simulink model "3Phase_Differential_Buck_Inverter"  (R2022b)
settings: Solver=VariableStepAuto  StartTime=0.0  StopTime=10.0  RelTol=1e-3
model workspace (MAT data in the model file):
  phi1 = 1.5991904307
  phi2 = 6.28
  phi3 = 3.23480337931
libraries: spsSeriesRLCBranchLib x9, spsGroundLib x7, spsMosfetLib x6, spsVoltageMeasurementLib x6, spsDCVoltageSourceLib x1, spsTriangleGeneratorLib x1, sps_lib x1
settings Model: Creator=nishi  LastModifiedBy=nishi

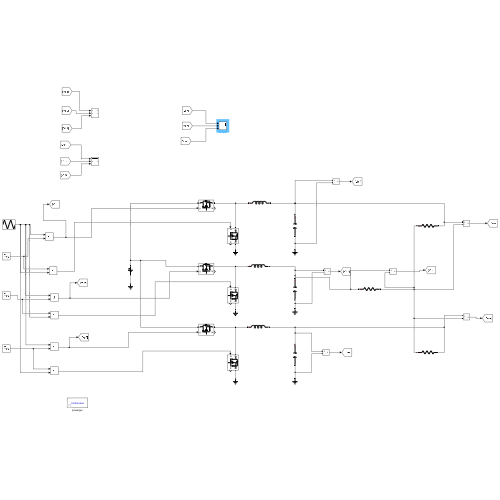
[thumbnail: Simulink's stored preview of the top-level diagram]
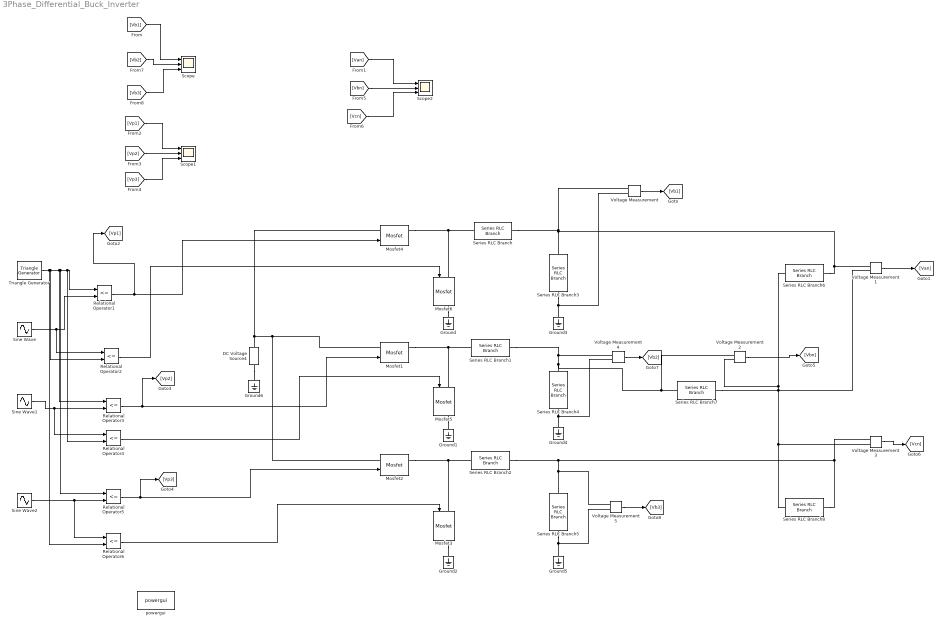
== system 3Phase_Differential_Buck_Inverter ==
  DC Voltage Source4 : spsDCVoltageSourceLib/DC Voltage Source  Amplitude=24  Measurements=None
  Ground{,1..6} (7 alike) : spsGroundLib/Ground  LConnTagsString=a
  Mosfet{1..6} (6 alike) : spsMosfetLib/Mosfet  Ron=1e-7  Lon=0  Rd=1e-10  Vfd=0  IC=0  Rs=inf  Cs=0  Measurements=on
  Relational Operator{1..6} (6 alike) : RelationalOperator  Operator=<=  OutDataTypeStr=boolean  RndMeth=Simplest  InputSameDT=off
  Scope : Scope  NumInputPorts=3
  Scope1 : Scope  NumInputPorts=3
  Scope2 : Scope  NumInputPorts=3
  Series RLC Branch : spsSeriesRLCBranchLib/Series RLC Branch  LConnTagsString=__new0  RConnTagsString=__new0  BranchType=L  Resistance=1  Inductance=3e-3  SetiL0=off  InitialCurrent=0  Capacitance=1e-6  Setx0=off  InitialVoltage=0  Measurements=None
  Series RLC Branch1 : spsSeriesRLCBranchLib/Series RLC Branch  LConnTagsString=__new0  RConnTagsString=__new0  BranchType=L  Resistance=1  Inductance=3e-3  SetiL0=off  InitialCurrent=0  Capacitance=1e-6  Setx0=off  InitialVoltage=0  Measurements=None
  Series RLC Branch2 : spsSeriesRLCBranchLib/Series RLC Branch  LConnTagsString=__new0  RConnTagsString=__new0  BranchType=L  Resistance=1  Inductance=3e-3  SetiL0=off  InitialCurrent=0  Capacitance=1e-6  Setx0=off  InitialVoltage=0  Measurements=None
  Series RLC Branch3 : spsSeriesRLCBranchLib/Series RLC Branch  LConnTagsString=__new0  RConnTagsString=__new0  BranchType=C  Resistance=1  Inductance=1e-3  SetiL0=off  InitialCurrent=0  Capacitance=100e-6  Setx0=off  InitialVoltage=0  Measurements=None
  Series RLC Branch4 : spsSeriesRLCBranchLib/Series RLC Branch  LConnTagsString=__new0  RConnTagsString=__new0  BranchType=C  Resistance=1  Inductance=1e-3  SetiL0=off  InitialCurrent=0  Capacitance=100e-6  Setx0=off  InitialVoltage=0  Measurements=None
  Series RLC Branch5 : spsSeriesRLCBranchLib/Series RLC Branch  LConnTagsString=__new0  RConnTagsString=__new0  BranchType=C  Resistance=1  Inductance=1e-3  SetiL0=off  InitialCurrent=0  Capacitance=100e-6  Setx0=off  InitialVoltage=0  Measurements=None
  Series RLC Branch6 : spsSeriesRLCBranchLib/Series RLC Branch  LConnTagsString=__new0  RConnTagsString=__new0  BranchType=R  Resistance=6  Inductance=1e-3  SetiL0=off  InitialCurrent=0  Capacitance=1e-6  Setx0=off  InitialVoltage=0  Measurements=None
  Series RLC Branch7 : spsSeriesRLCBranchLib/Series RLC Branch  LConnTagsString=__new0  RConnTagsString=__new0  BranchType=R  Resistance=6  Inductance=1e-3  SetiL0=off  InitialCurrent=0  Capacitance=1e-6  Setx0=off  InitialVoltage=0  Measurements=None
  Series RLC Branch8 : spsSeriesRLCBranchLib/Series RLC Branch  LConnTagsString=__new0  RConnTagsString=__new0  BranchType=R  Resistance=6  Inductance=1e-3  SetiL0=off  InitialCurrent=0  Capacitance=1e-6  Setx0=off  InitialVoltage=0  Measurements=None
  Sine Wave : Sin  Frequency=314.16  SampleTime=0
  Sine Wave1 : Sin  Frequency=314.16  Phase=-2.094  SampleTime=0
  Sine Wave2 : Sin  Frequency=314.16  Phase=2.094  SampleTime=0
  Triangle Generator : spsTriangleGeneratorLib/Triangle Generator  Freq=20000  Phase=90  Ts=0
  Voltage Measurement{,1..5} (6 alike) : spsVoltageMeasurementLib/Voltage Measurement  PhasorSimulation=off  OutputType=Complex  PSBequivalent=0
  powergui : sps_lib/powergui  Priority=1  SimulationMode=Continuous  SampleTime=1e-6  frequency=60  Iterations=50  frequencyindice=0  Pbase=100e6  ErrMax=1e-4  UnitsV=kV  UnitsW=MW  buscounter=0  FunctionMessages=off  echomessages=off  EnableUseOfTLC=off  CurrentSourceSwitches=off  DisableSnubberDevices=off  DisableRonSwitches=off  DisableVfSwitches=off  DisplayEquations=off  AutomaticDiscreteSolvers=off  SolverType=Tustin/Backward Euler (TBE)  Interpol=off  ExternalGateDelay=off  methode=off  Ts=100  x0status=blocks  SPID=on  SwTol=0  HookPort=off  NonlinearTolerance=1e-4  nMaxIteration=100  ContinueOnMaxIteration=off  RestoreLinks=warning  ResistiveCurrentMeasurement=off  Frange=[0:2:500]  Ylog=off  Xlog=on  ShowGrid=off  save=off  variable=ZData  structure=0  ZoomFFT=off  StartTime=0.0  cycles=1  DisplayStyle=1  fundamental=60  FreqAxis=off  MaxFrequency=1000  frequencyindicesteady=1  RmsSteady=1  display=off
  wires:
  Voltage Measurement/1 -> [Vb1]
  Voltage Measurement1/1 -> [Van]
  [Vb1] -> Scope/1
  Triangle Generator/1 -> Relational Operator6/2, Relational Operator2/2, Relational Operator5/1, Relational Operator4/2, Relational Operator1/1, Relational Operator3/1
  Sine Wave/1 -> Relational Operator2/1, Relational Operator1/2
  Relational Operator1/1 -> [Vp1], Mosfet4/1
  Relational Operator2/1 -> Mosfet6/1
  Sine Wave1/1 -> Relational Operator4/1, Relational Operator3/2
  Relational Operator3/1 -> [Vp2], Mosfet1/1
  Relational Operator4/1 -> Mosfet5/1
  Sine Wave2/1 -> Relational Operator6/1, Relational Operator5/2
  Relational Operator5/1 -> [Vp3], Mosfet2/1
  Relational Operator6/1 -> Mosfet3/1
  [Vp1] -> Scope1/1
  [Vp2] -> Scope1/2
  [Vp3] -> Scope1/3
  Voltage Measurement2/1 -> [Vbn]
  Voltage Measurement3/1 -> [Vcn]
  [Van] -> Scope2/1
  [Vbn] -> Scope2/2
  [Vcn] -> Scope2/3
  Voltage Measurement4/1 -> [Vb2]
  Voltage Measurement5/1 -> [Vb3]
  [Vb2] -> Scope/2
  [Vb3] -> Scope/3
  connections:
  Mosfet4/RConn1 -- Mosfet6/LConn1 -- Series RLC Branch/LConn1
  Mosfet6/RConn1 -- Ground/LConn1
  Mosfet1/RConn1 -- Mosfet5/LConn1 -- Series RLC Branch1/LConn1
  Mosfet5/RConn1 -- Ground1/LConn1
  Mosfet2/RConn1 -- Mosfet3/LConn1 -- Series RLC Branch2/LConn1
  Mosfet3/RConn1 -- Ground2/LConn1
  Series RLC Branch/RConn1 -- Voltage Measurement1/LConn1 -- Series RLC Branch6/RConn1 -- Series RLC Branch3/LConn1 -- Voltage Measurement/LConn1
  Series RLC Branch1/RConn1 -- Voltage Measurement4/LConn1 -- Voltage Measurement2/LConn1 -- Series RLC Branch7/LConn1 -- Series RLC Branch4/LConn1
  Series RLC Branch2/RConn1 -- Voltage Measurement3/LConn1 -- Series RLC Branch8/RConn1 -- Voltage Measurement5/LConn1 -- Series RLC Branch5/LConn1
  Series RLC Branch3/RConn1 -- Voltage Measurement/LConn2 -- Ground3/LConn1
  Series RLC Branch4/RConn1 -- Voltage Measurement4/LConn2 -- Ground4/LConn1
  Series RLC Branch5/RConn1 -- Ground5/LConn1 -- Voltage Measurement5/LConn2
  DC Voltage Source4/LConn1 -- Ground6/LConn1
  DC Voltage Source4/RConn1 -- Mosfet2/LConn1 -- Mosfet1/LConn1 -- Mosfet4/LConn1
  Series RLC Branch6/LConn1 -- Voltage Measurement2/LConn2 -- Voltage Measurement1/LConn2 -- Series RLC Branch7/RConn1 -- Voltage Measurement3/LConn2 -- Series RLC Branch8/LConn1
